simulink model "sl_opspace"  (R2015a)
settings: Solver=ode45  StartTime=0.0  StopTime=2  RelTol=1e-3
InitFcn:
  | fprintf('parameters initialized in InitFcn\n');
  | 
  | mdl_puma560
  | 
  | q = [0 pi/4 pi 0 -pi/4 0];
  | TE = p560.fkine(q);
  | Sf = TE.R
  | 
  | % edit next 2 lines to change compliant motion axes
  | %  1 = freespace controlled motion
  | %  0 = constrained compliant motion
  | 
  | sigma_f = diag([1 1 0]);  % translation
  | sigma_t = diag([1 1 1]);  % rotation
  | 
  | 
  | 
  | omega = blkdiag( Sf'*sigma_f*Sf, Sf'*sigma_t*Sf)
  | omega_tilde = blkdiag( Sf'*(eye(3,3)-sigma_f)*Sf, Sf'*(eye(3,3)-sigma_t)*Sf)
undefined symbols (not defined in the file): cinertia, nofriction, p560, qn, transl, troty
libraries: roblocks x6
settings Model: Creator=corkep  LastModifiedBy=corkep
settings DataIOCC: ReturnWorkspaceOutputs=on  TimeSaveName=t  OutputSaveName=y  ReturnWorkspaceOutputsName=opspace
settings HardwareCC: ProdBitPerPointer=64  ProdLargestAtomicFloat=Float  ProdIntDivRoundTo=Zero  ProdEndianess=LittleEndian  ProdHWDeviceType=Specified
settings GRTTargetCC: GeneratePreprocessorConditionals=Use local settings

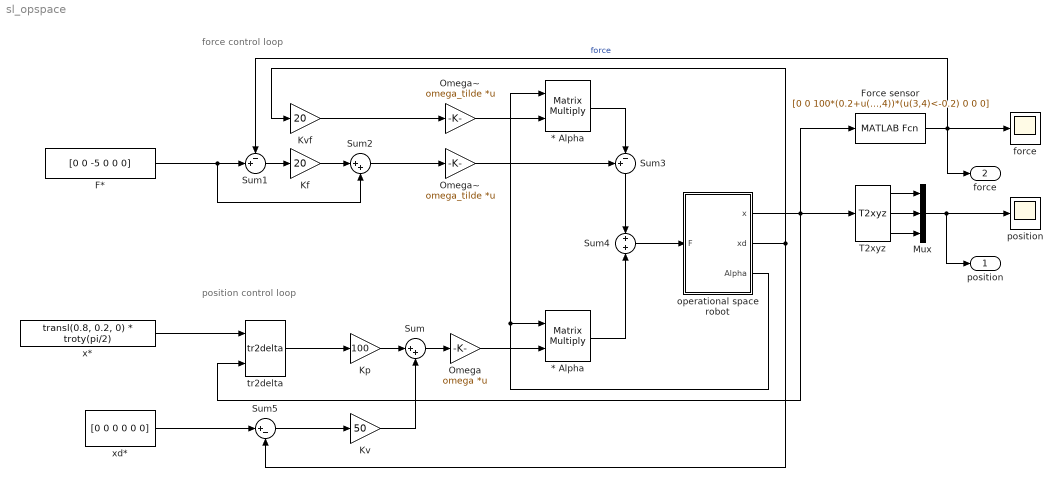
== system sl_opspace ==
  note: position control loop
  note: force control loop
  * Alpha : Product  Multiplication=Matrix(*)
  "* Alpha " : Product  Multiplication=Matrix(*)
  F* : Constant  Value=[0 0 -5 0 0 0]
  Force sensor : MATLABFcn  MATLABFcn=[0 0 100*(0.2+u(3,4))*(u(3,4)<-0.2) 0 0 0]
  Kf : Gain  Gain=20
  Kp : Gain  Gain=100
  Kv : Gain  Gain=50
  Kvf : Gain  Gain=20
  Mux : Mux  Inputs=3
  Omega : Gain  Gain=omega  Multiplication=Matrix(K*u)
  Omega~ : Gain  Gain=omega_tilde  Multiplication=Matrix(K*u)
  "Omega~ " : Gain  Gain=omega_tilde  Multiplication=Matrix(K*u)
  Sum : Sum  Inputs=|++
  Sum1 : Sum  Inputs=-+|
  Sum2 : Sum  Inputs=|++
  Sum3 : Sum  Inputs=+-|
  Sum4 : Sum  Inputs=+|+
  Sum5 : Sum  Inputs=|+-
  T2xyz : roblocks/Toolbox/T2xyz
  force : Scope
      settings: TimeRange=auto  ShowLegends=on  MaxDataPoints=5000  SaveToWorkspace=off  SaveName=ScopeData2  YMin=-6.57693  YMax=0.73077  SampleTime=-1
  operational space robot : Subsystem  mask{robot=nofriction(p560), q0=qn}
      mask prompts: q0 "Initial joint angles"
  position : Scope
      settings: TimeRange=auto  ShowLegends=on  MaxDataPoints=5000  SaveToWorkspace=off  SaveName=ScopeData  YMin=-0.3901  YMax=0.92625  SampleTime=-1
  tr2delta : roblocks/Toolbox/tr2delta
  x* : Constant  Value=transl(0.8, 0.2, 0) * troty(pi/2)
  xd* : Constant  Value=[0 0 0 0 0 0]
  "position " : Outport
  "force " : Outport  Port=2
  wires:
  x*/1 -> tr2delta/1
  operational space robot/1(x) -> T2xyz/1, Force sensor/1, tr2delta/2
  operational space robot/3(Alpha) -> * Alpha/1, "* Alpha "/1
  Sum/1 -> Omega/1
  Kp/1 -> Sum/1
  tr2delta/1 -> Kp/1
  Kv/1 -> Sum/2
  operational space robot/2(xd) -> Kvf/1, Sum5/2
  Force sensor/1 -> "force "/1, force/1, Sum1/1  "force"
  F*/1 -> Sum2/2, Sum1/2
  Sum1/1 -> Kf/1
  Kf/1 -> Sum2/1
  Kvf/1 -> Omega~/1
  Sum2/1 -> "Omega~ "/1
  Omega~/1 -> * Alpha/2
  * Alpha/1 -> Sum3/2
  "Omega~ "/1 -> Sum3/1
  Sum3/1 -> Sum4/1
  "* Alpha "/1 -> Sum4/2
  Omega/1 -> "* Alpha "/2
  xd*/1 -> Sum5/1
  Sum5/1 -> Kv/1
  Sum4/1 -> operational space robot/1(F)
  T2xyz/1 -> Mux/1
  T2xyz/2 -> Mux/2
  T2xyz/3 -> Mux/3
  Mux/1 -> "position "/1, position/1

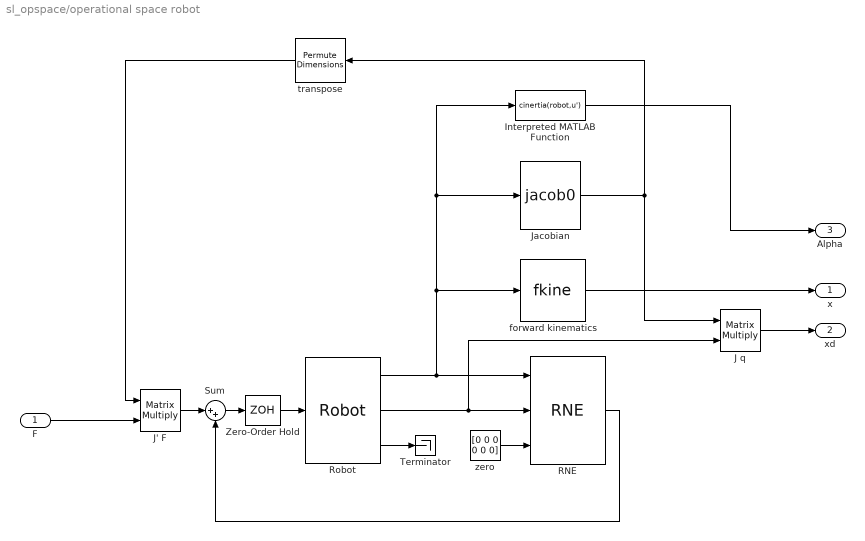
== system sl_opspace/operational space robot ==
  F : Inport
  Interpreted MATLAB Function : MATLABFcn  MATLABFcn=cinertia(robot,u')  OutputDimensions=[6 6]  Output1D=off
  J q : Product  Multiplication=Matrix(*)
  J' F : Product  Multiplication=Matrix(*)
  Jacobian : roblocks/Arm/jacob0   robot=robot
  RNE : roblocks/Arm/RNE  robot=robot  grav=[0 0 9.81]
  Robot : roblocks/Arm/Robot  robot=robot  q0=q0
  Sum : Sum  Inputs=|++
  Terminator : Terminator
  Zero-Order Hold : ZeroOrderHold  SampleTime=5e-3
  forward kinematics : roblocks/Arm/fkine  robot=robot
  transpose : PermuteDimensions
  zero : Constant  Value=[0 0 0 0 0 0]
  x : Outport
  xd : Outport  Port=2
  Alpha : Outport  Port=3
  wires:
  Interpreted MATLAB Function/1 -> Alpha/1
  Zero-Order Hold/1 -> Robot/1
  Sum/1 -> Zero-Order Hold/1
  F/1 -> J' F/2
  transpose/1 -> J' F/1
  J' F/1 -> Sum/1
  RNE/1 -> Sum/2
  zero/1 -> RNE/3
  Robot/3 -> Terminator/1
  Robot/2 -> RNE/2, J q/2
  Robot/1 -> RNE/1, forward kinematics/1, Interpreted MATLAB Function/1, Jacobian/1
  forward kinematics/1 -> x/1
  J q/1 -> xd/1
  Jacobian/1 -> transpose/1, J q/1
